simulink model "Robotesic_model"  (R2021b)
settings: Solver=ode4  StartTime=0.0  StopTime=100  FixedStep=0.001  RelTol=1e-3
values from neighbouring files (symbols this model uses):
  I11 = m*L*L*(4/3+mu1+mu2)    (= 28.3333333333)    [ROBOTICS_2021.m]
  I21 = m*L*L*(1/2+mu2)    (= 26.25)    [ROBOTICS_2021.m]
  I22 = m*L*L*(1/3+mu2)    (= 25.8333333333)    [ROBOTICS_2021.m]
  mu = 10    [ROBOTICS_2021.m]
  mu1 = 0.0    (= 0)    [ROBOTICS_2021.m]
  tao = 1    [ROBOTICS_2021.m]
  wn = 1    [ROBOTICS_2021.m]
settings Model: Creator=DELL  LastModifiedBy=Lenovo
settings SolverCC: AlgebraicLoopSolver=TrustRegion
settings DataIOCC: ReturnWorkspaceOutputs=off
settings DebuggingCC: SFMachineParentedDataDiag=warning  ArithmeticOperatorsInVariantConditions=warning
settings SFSimCC: SimUseLocalCustomCode=off  CustomCodeUndefinedFunction=UseInterfaceOnly
settings RTWCC: RTWUseLocalCustomCode=off
settings CodeAppCC: StateflowObjectComments=on

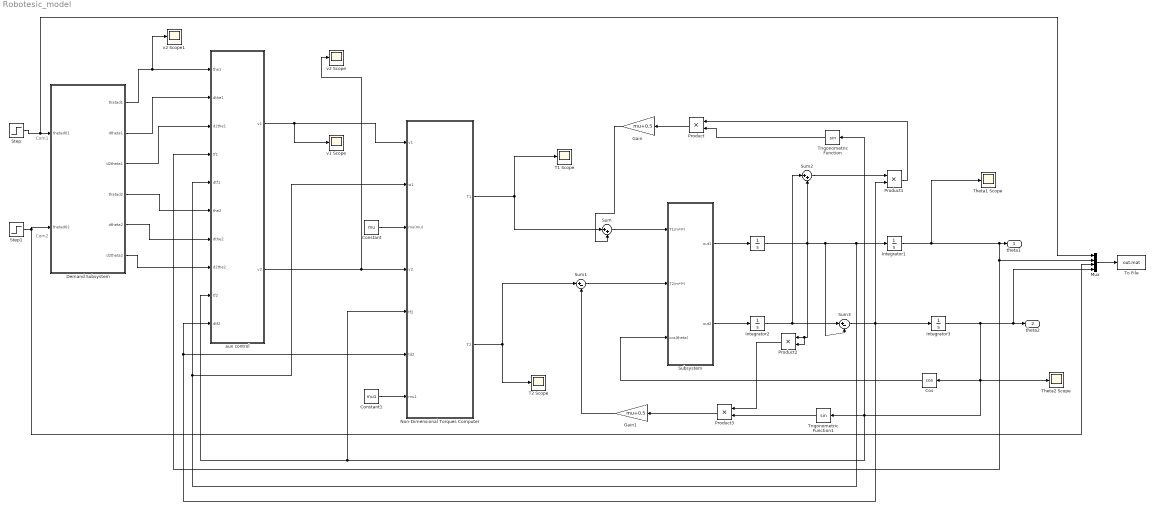
== system Robotesic_model ==
  note: Com1
  note: Com2
  " " : Integrator
  Constant : Constant  Value=mu
  Constant1 : Constant  Value=mu1
  Cos : Trigonometry  Operator=cos
  Demand Subsystem : Subsystem
  Gain : Gain  Gain=mu+0.5
  Gain1 : Gain  Gain=mu+0.5
  Integrator1 : Integrator  InitialCondition=6.87*pi/180*0
  Integrator2 : Integrator
  Integrator3 : Integrator
  Mux : Mux
  Non-Dimensional Torques Computer : Subsystem
  Product{,1..3} (4 alike) : Product
  Step : Step  Time=0  After=6.87*pi/180*0  SampleTime=0
  Step1 : Step  Time=0  After=240*pi/180*1  SampleTime=0
  Subsystem : Subsystem
  Sum : Sum  Inputs=|++
  Sum1 : Sum  Inputs=|+-
  Sum2 : Sum  Inputs=|++
  Sum3 : Sum  Inputs=|+-
  T1 Scope : Scope
  T2 Scope : Scope
  Theta1 Scope : Scope
  Theta2 Scope : Scope
  To File : ToFile  Filename=out.mat  MatrixName=y
  Trigonometric Function : Trigonometry
  Trigonometric Function1 : Trigonometry
  aux control : Subsystem
  v1 Scope : Scope
  v2 Scope : Scope
  v2 Scope1 : Scope
  theta1 : Outport
  theta2 : Outport  Port=2
  wires:
  Demand Subsystem/1(thatad1) -> v2 Scope1/1, aux control/1(the1)
  Demand Subsystem/2(dtheta1) -> aux control/2(dthe1)
  Demand Subsystem/3(d2theta1) -> aux control/3(d2the1)
  Demand Subsystem/4(thatad2) -> aux control/6(the2)
  Demand Subsystem/5(dtheta2) -> aux control/7(dthe2)
  Demand Subsystem/6(d2theta2) -> aux control/8(d2the2)
  aux control/1(v1) -> v1 Scope/1, Non-Dimensional Torques Computer/1(v1)
  aux control/2(v2) -> v2 Scope/1, Non-Dimensional Torques Computer/4(v2)
  Non-Dimensional Torques Computer/1(T1) -> Sum/1, T1 Scope/1
  Sum/1 -> Subsystem/1(T1/m*I*I)
  Sum1/1 -> Subsystem/2(T2/m*I*I)
  Non-Dimensional Torques Computer/2(T2) -> Sum1/1, T2 Scope/1
  Product/1 -> Gain/1
  Gain/1 -> Sum/2
  Trigonometric Function/1 -> Product/2
  Sum2/1 -> Product1/1
  Integrator1/1 -> Theta1 Scope/1, Mux/2, aux control/4(tf1), theta1/1
  " "/1 -> Sum2/2, Non-Dimensional Torques Computer/2(w1), aux control/5(dtf1), Integrator1/1, Sum3/2, Product2/1, Product2/2
  Subsystem/1(out1) -> " "/1
  Subsystem/2(out2) -> Integrator2/1
  Integrator2/1 -> Sum3/1, Sum2/1
  Product1/1 -> Product/1
  Gain1/1 -> Sum1/2
  Product3/1 -> Gain1/1
  Product2/1 -> Product3/1
  Trigonometric Function1/1 -> Product3/2
  Cos/1 -> Subsystem/3(cos(theta))
  Integrator3/1 -> Mux/4, theta2/1, Theta2 Scope/1, aux control/9(tf2), Non-Dimensional Torques Computer/5(tf2), Trigonometric Function/1, Trigonometric Function1/1, Cos/1
  Sum3/1 -> aux control/10(dtf2), Non-Dimensional Torques Computer/6(td2), Product1/2, Integrator3/1
  Constant1/1 -> Non-Dimensional Torques Computer/7(mu1)
  Constant/1 -> Non-Dimensional Torques Computer/3(mu(mu))
  Mux/1 -> To File/1
  Step/1 -> Mux/1, Demand Subsystem/1(thetad01)
  Step1/1 -> Mux/3, Demand Subsystem/2(thetad02)

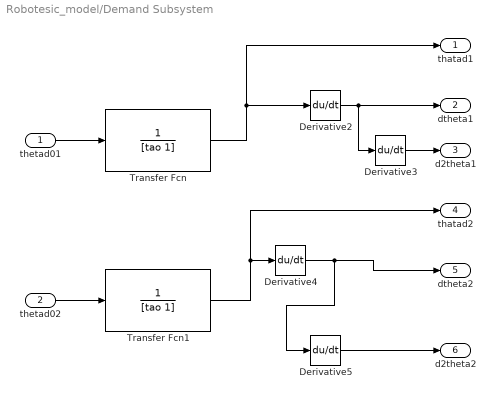
== system Robotesic_model/Demand Subsystem ==
  thetad01 : Inport
  thetad02 : Inport  Port=2
  Derivative{2..5} (4 alike) : Derivative
  Transfer Fcn : TransferFcn  Denominator=[tao 1]
  Transfer Fcn1 : TransferFcn  Denominator=[tao 1]
  thatad1 : Outport
  dtheta1 : Outport  Port=2
  d2theta1 : Outport  Port=3
  thatad2 : Outport  Port=4
  dtheta2 : Outport  Port=5
  d2theta2 : Outport  Port=6
  wires:
  Transfer Fcn/1 -> Derivative2/1, thatad1/1
  Transfer Fcn1/1 -> Derivative4/1, thatad2/1
  Derivative3/1 -> d2theta1/1
  thetad01/1 -> Transfer Fcn/1
  thetad02/1 -> Transfer Fcn1/1
  Derivative2/1 -> Derivative3/1, dtheta1/1
  Derivative4/1 -> Derivative5/1, dtheta2/1
  Derivative5/1 -> d2theta2/1

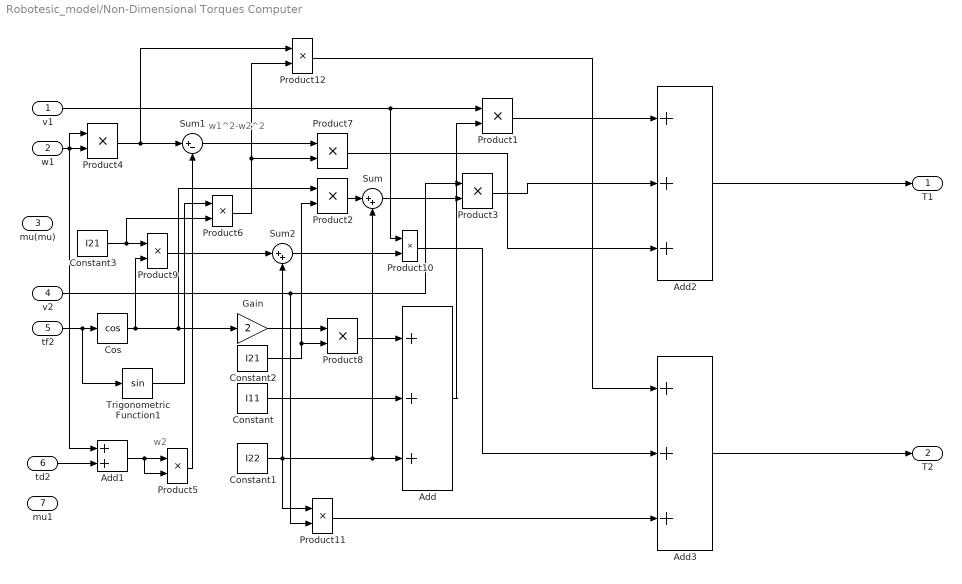
== system Robotesic_model/Non-Dimensional Torques Computer ==
  note: w1^2-w2^2
  note: w2
  v1 : Inport
  w1 : Inport  Port=2
  mu(mu) : Inport  Port=3
  v2 : Inport  Port=4
  tf2 : Inport  Port=5
  td2 : Inport  Port=6
  mu1 : Inport  Port=7
  Add : Sum  Inputs=+++
  Add1 : Sum
  Add2 : Sum  Inputs=+++
  Add3 : Sum  Inputs=+++
  Constant : Constant  Value=I11
  Constant1 : Constant  Value=I22
  Constant2 : Constant  Value=I21
  Constant3 : Constant  Value=I21
  Cos : Trigonometry  Operator=cos
  Gain : Gain  Gain=2
  Product{1..12} (12 alike) : Product
  Sum : Sum  Inputs=|++
  Sum1 : Sum  Inputs=|+-
  Sum2 : Sum  Inputs=|++
  Trigonometric Function1 : Trigonometry
  T1 : Outport
  T2 : Outport  Port=2
  wires:
  tf2/1 -> Cos/1, Trigonometric Function1/1
  Cos/1 -> Product9/2, Product2/1, Gain/1
  Constant/1 -> Add/2
  Constant1/1 -> Product11/1, Sum2/2, Add/3, Sum/2
  v1/1 -> Product10/1, Product1/1
  Add/1 -> Product1/2
  v2/1 -> Product11/2, Product3/1
  Product2/1 -> Sum/1
  Sum/1 -> Product3/2
  w1/1 -> Add1/1, Product4/1, Product4/2
  td2/1 -> Add1/2
  Add1/1 -> Product5/2, Product5/1
  Product4/1 -> Product12/1, Sum1/1
  Product5/1 -> Sum1/2
  Sum1/1 -> Product7/1
  Trigonometric Function1/1 -> Product6/1
  Product6/1 -> Product7/2, Product12/2
  Product3/1 -> Add2/2
  Product7/1 -> Add2/3
  Product1/1 -> Add2/1
  Add2/1 -> T1/1
  Product8/1 -> Add/1
  Gain/1 -> Product8/1
  Constant2/1 -> Product2/2, Product8/2
  Constant3/1 -> Product6/2, Product9/1
  Product9/1 -> Sum2/1
  Sum2/1 -> Product10/2
  Product11/1 -> Add3/3
  Product10/1 -> Add3/2
  Product12/1 -> Add3/1
  Add3/1 -> T2/1

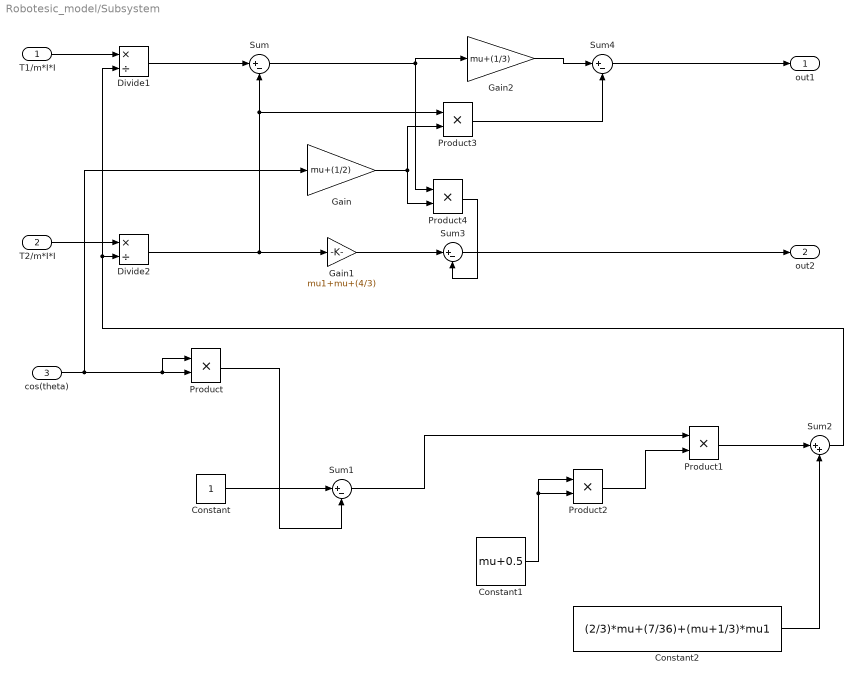
== system Robotesic_model/Subsystem ==
  T1/m*I*I : Inport
  T2/m*I*I : Inport  Port=2
  cos(theta) : Inport  Port=3
  Constant : Constant
  Constant1 : Constant  Value=mu+0.5
  Constant2 : Constant  Value=(2/3)*mu+(7/36)+(mu+1/3)*mu1
  Divide1 : Product  Inputs=*/
  Divide2 : Product  Inputs=*/
  Gain : Gain  Gain=mu+(1/2)
  Gain1 : Gain  Gain=mu1+mu+(4/3)
  Gain2 : Gain  Gain=mu+(1/3)
  Product{,1..4} (5 alike) : Product
  Sum{,1,3..4} (4 alike) : Sum  Inputs=|+-
  Sum2 : Sum  Inputs=|++
  out1 : Outport
  out2 : Outport  Port=2
  wires:
  T1/m*I*I/1 -> Divide1/1
  Divide1/1 -> Sum/1
  T2/m*I*I/1 -> Divide2/1
  cos(theta)/1 -> Gain/1, Product/1, Product/2
  Constant/1 -> Sum1/1
  Product/1 -> Sum1/2
  Sum1/1 -> Product1/1
  Constant1/1 -> Product2/2, Product2/1
  Product2/1 -> Product1/2
  Product1/1 -> Sum2/1
  Constant2/1 -> Sum2/2
  Sum2/1 -> Divide1/2, Divide2/2
  Divide2/1 -> Product3/1, Sum/2, Gain1/1
  Sum/1 -> Product4/1, Gain2/1
  Gain/1 -> Product3/2, Product4/2
  Gain1/1 -> Sum3/1
  Sum3/1 -> out2/1
  Product4/1 -> Sum3/2
  Gain2/1 -> Sum4/1
  Sum4/1 -> out1/1
  Product3/1 -> Sum4/2

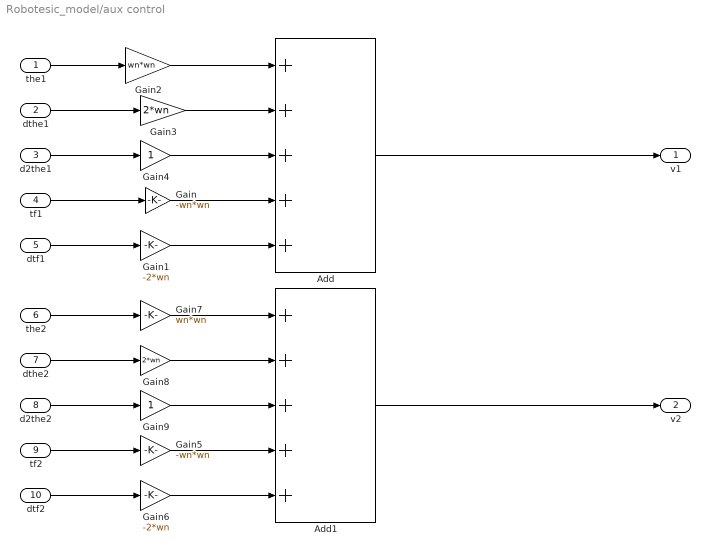
== system Robotesic_model/aux control ==
  the1 : Inport
  dthe1 : Inport  Port=2
  d2the1 : Inport  Port=3
  tf1 : Inport  Port=4
  dtf1 : Inport  Port=5
  the2 : Inport  Port=6
  dthe2 : Inport  Port=7
  d2the2 : Inport  Port=8
  tf2 : Inport  Port=9
  dtf2 : Inport  Port=10
  Add : Sum  Inputs=+++++
  Add1 : Sum  Inputs=+++++
  Gain : Gain  Gain=-wn*wn
  Gain1 : Gain  Gain=-2*wn
  Gain2 : Gain  Gain=wn*wn
  Gain3 : Gain  Gain=2*wn
  Gain4 : Gain
  Gain5 : Gain  Gain=-wn*wn
  Gain6 : Gain  Gain=-2*wn
  Gain7 : Gain  Gain=wn*wn
  Gain8 : Gain  Gain=2*wn
  Gain9 : Gain
  v1 : Outport
  v2 : Outport  Port=2
  wires:
  tf1/1 -> Gain/1
  dtf1/1 -> Gain1/1
  the1/1 -> Gain2/1
  dthe1/1 -> Gain3/1
  d2the1/1 -> Gain4/1
  Gain2/1 -> Add/1
  Gain3/1 -> Add/2
  Gain4/1 -> Add/3
  Gain/1 -> Add/4
  Gain1/1 -> Add/5
  Add/1 -> v1/1
  Gain8/1 -> Add1/2
  Add1/1 -> v2/1
  Gain6/1 -> Add1/5
  d2the2/1 -> Gain9/1
  tf2/1 -> Gain5/1
  Gain9/1 -> Add1/3
  Gain5/1 -> Add1/4
  dtf2/1 -> Gain6/1
  the2/1 -> Gain7/1
  dthe2/1 -> Gain8/1
  Gain7/1 -> Add1/1
